simulink model "previous_plan_simulator"  (R2024b)
settings: Solver=VariableStepAuto  StartTime=0.0  StopTime=10.0  RelTol=1e-3
values from neighbouring files (symbols this model uses):
  final_point_cm = [1; 5; 3]    [previous_plan.m]
  init_point_cm = [2; 0; 7]    [previous_plan.m]
settings Model: Creator=zhes  LastModifiedBy=zhes

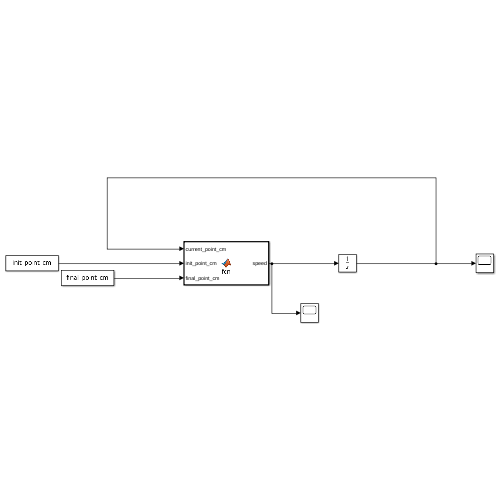
[thumbnail: Simulink's stored preview of the top-level diagram]
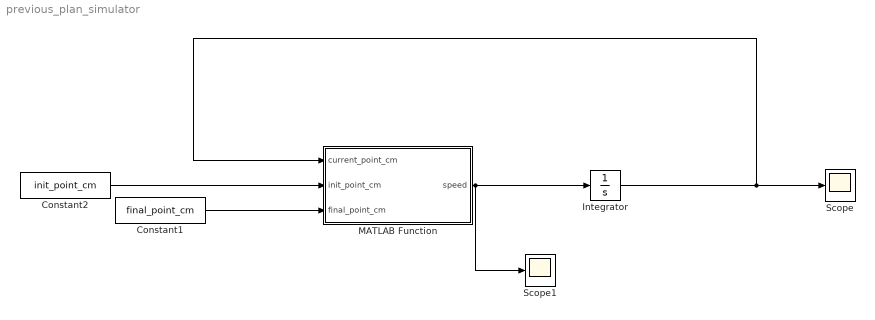
== system previous_plan_simulator ==
  Constant1 : Constant  Value=final_point_cm
  Constant2 : Constant  Value=init_point_cm
  Integrator : Integrator  InitialCondition=init_point_cm
  MATLAB Function : MATLAB Function  TreatAsAtomicUnit=on
  Scope : Scope
  Scope1 : Scope
  wires:
  Integrator/1 -> Scope/1, MATLAB Function/1(current_point_cm)
  Constant1/1 -> MATLAB Function/3(final_point_cm)
  Constant2/1 -> MATLAB Function/2(init_point_cm)
  MATLAB Function/1(speed) -> Scope1/1, Integrator/1

== matlab function previous_plan_simulator/MATLAB Function ==
  data: current_point_cm input; init_point_cm input; speed output; final_point_cm input
function speed = fcn(current_point_cm,init_point_cm,final_point_cm)

MaxSpeed = 1000;

CMS_FOR_10_REVOLUTIONS = 60;
CM_PER_REVOLUTION = CMS_FOR_10_REVOLUTIONS / 10;
STEPS_PER_CM = 800 / CM_PER_REVOLUTION;

%%
reverseKinematics = @(x,y,z) [x + y; x - y; x - y + z] * STEPS_PER_CM;

%
init_step = init_point_cm;

current_step = current_point_cm;
final_step = final_point_cm;

%
motor_current = reverseKinematics(current_step(1), current_step(2), current_step(3));
motor_final = reverseKinematics(final_step(1), final_step(2), final_step(3));

%
delta_motor = motor_final - motor_current;

%
abs_x = abs(delta_motor(1));
abs_y = abs(delta_motor(2));
abs_z = abs(delta_motor(3));

%
max_distance = max([abs_x, abs_y, abs_z]);

%
x_ratio = abs_x / max_distance;
y_ratio = abs_y / max_distance;
z_ratio = abs_z / max_distance;

%
x_speed = x_ratio * MaxSpeed * sign(delta_motor(1));
y_speed = y_ratio * MaxSpeed * sign(delta_motor(2));
z_speed = z_ratio * MaxSpeed * sign(delta_motor(3));


speed = [x_speed; y_speed; z_speed];
